simulink model "tricopter_control"  (R2018a)
settings: Solver=VariableStepAuto  StartTime=0.0  StopTime=100  RelTol=1e-3
settings Model: Creator=Aniruddh  LastModifiedBy=Aniruddh

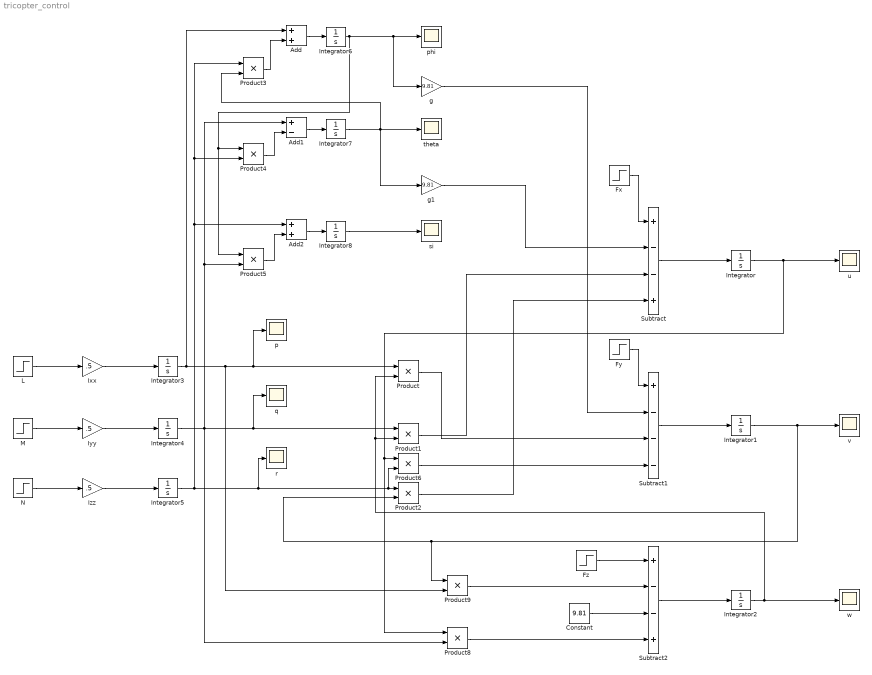
== system tricopter_control ==
  Add : Sum
  Add1 : Sum  Inputs=+-
  Add2 : Sum
  Constant : Constant  Value=9.81
  Fx : Step  Time=3  SampleTime=0
  Fy : Step  Time=3  After=0  SampleTime=0
  Fz : Step  Time=3  After=.5  SampleTime=0
  Integrator : Integrator
  Integrator1 : Integrator
  Integrator2 : Integrator
  Integrator3 : Integrator  LimitOutput=on  UpperSaturationLimit=.1  LowerSaturationLimit=0
  Integrator4 : Integrator  LimitOutput=on  UpperSaturationLimit=.1  LowerSaturationLimit=0
  Integrator5 : Integrator  LimitOutput=on  UpperSaturationLimit=.5  LowerSaturationLimit=0
  Integrator6 : Integrator  LimitOutput=on  UpperSaturationLimit=2  LowerSaturationLimit=0
  Integrator7 : Integrator  LimitOutput=on  UpperSaturationLimit=2  LowerSaturationLimit=0
  Integrator8 : Integrator  LimitOutput=on  UpperSaturationLimit=2  LowerSaturationLimit=0
  Ixx : Gain  Gain=.5
  Iyy : Gain  Gain=.5
  Izz : Gain  Gain=.5
  L : Step  Time=3  After=.1  SampleTime=0
  M : Step  Time=3  After=.1  SampleTime=0
  N : Step  Time=3  After=.1  SampleTime=0
  Product{,1..6,8..9} (9 alike) : Product
  Subtract : Sum  Inputs=+--+
  Subtract1 : Sum  Inputs=+---
  Subtract2 : Sum  Inputs=+--+
  g : Gain  Gain=9.81
  g1 : Gain  Gain=9.81
  p : Scope
  phi : Scope
  q : Scope
  r : Scope
  si : Scope
  theta : Scope
  u : Scope
  v : Scope
  w : Scope
  wires:
  Integrator/1 -> Product8/1, Product6/1, u/1
  Subtract/1 -> Integrator/1
  Fx/1 -> Subtract/1
  Subtract1/1 -> Integrator1/1
  Integrator1/1 -> Product9/1, Product2/2, v/1
  Subtract2/1 -> Integrator2/1
  Integrator2/1 -> Product/2, Product1/2, w/1
  L/1 -> Ixx/1
  M/1 -> Iyy/1
  N/1 -> Izz/1
  Ixx/1 -> Integrator3/1
  Iyy/1 -> Integrator4/1
  Izz/1 -> Integrator5/1
  Integrator3/1 -> Add/1, Product9/2, p/1, Product/1
  Integrator5/1 -> Add2/1, Product4/2, Product3/1, r/1, Product6/2, Product2/1
  Integrator4/1 -> Product8/2, Add1/1, Product5/2, q/1, Product1/1
  Fy/1 -> Subtract1/1
  Fz/1 -> Subtract2/1
  Product2/1 -> Subtract/4
  Product1/1 -> Subtract/3
  Add/1 -> Integrator6/1
  Add1/1 -> Integrator7/1
  Add2/1 -> Integrator8/1
  Integrator7/1 -> g1/1, theta/1, Product3/2
  Product3/1 -> Add/2
  Product5/1 -> Add2/2
  Product4/1 -> Add1/2
  g1/1 -> Subtract/2
  Integrator8/1 -> si/1
  Integrator6/1 -> Product5/1, Product4/1, g/1, phi/1
  Constant/1 -> Subtract2/3
  g/1 -> Subtract1/2
  Product/1 -> Subtract1/3
  Product6/1 -> Subtract1/4
  Product8/1 -> Subtract2/4
  Product9/1 -> Subtract2/2
